simulink model "controllo_Completo_v14"  (R2025a)
settings: Solver=VariableStepAuto  StartTime=0.0  StopTime=Durata_Simulazione  MaxStep=Passo_integrazione_massimo  RelTol=1e-3
values from neighbouring files (symbols this model uses):
  C_bat_eq_rx = 1.0    (= 1)    [p_schema_completo_generale_v2.m]
  C_bat_eq_tx = 3.5    [p_schema_completo_generale_v2.m]
  C_bus_dc_dc = 1.5e-3    (= 0.0015)    [p_schema_completo_generale_v2.m]
  C_ris = 1/(w_dc_ac_nom^2*L_coil)    (= 6.49245057301e-08)    [p_schema_completo_generale_v2.m]
  dead_time_dc_dc = 0.3e-6    (= 3e-07)    [p_schema_completo_generale_v2.m]
  duty_A_0_tx = V_bat_0_tx/V_dc_0_tx    (= 0.472727272727)    [p_schema_completo_generale_v2.m]
  duty_B_0_tx = duty_A_0_tx    (= 0.472727272727)    [p_schema_completo_generale_v2.m]
  duty_leg_A_dc_dc_0_tx = V_bat_0_tx/V_dc_0_tx    (= 0.472727272727)    [p_schema_completo_generale_v2.m]
  duty_leg_B_dc_dc_0_tx = duty_leg_A_dc_dc_0_tx    (= 0.472727272727)    [p_schema_completo_generale_v2.m]
  Ibat_rif_max = 50    [p_schema_completo_generale_v2.m]
  Ibat_rif_min = -50    [p_schema_completo_generale_v2.m]
  Kp_P_tensione_batteria_rx = 1/modulo_catena_aperta_tensione_batteria_reg_P_rx    [p_schema_completo_generale_v2.m]
  Kp_P_tensione_batteria_tx = 1/modulo_catena_aperta_tensione_batteria_reg_P_tx    [p_schema_completo_generale_v2.m]
  L_coil = 54e-6    (= 5.4e-05)    [p_schema_completo_generale_v2.m]
  L_filtro_dc_dc = 65e-6    (= 6.5e-05)    [p_schema_completo_generale_v2.m]
  M_coil = k*sqrt(L_coil^2)    [p_schema_completo_generale_v2.m]
  Parametri_Controllori = [Parametri_Controllori     PI_corrente_trasm_tf_disc_den(2) PI_corrente_trasm_tf_disc_num(1) PI_corrente_trasm_tf_disc_num(2)]    [p_schema_completo_generale_v2.m]
  R_bat = 32e-3    (= 0.032)    [p_schema_completo_generale_v2.m]
  R_coil = w_dc_ac_nom*L_coil/Q_coil    (= 0.2883982056)    [p_schema_completo_generale_v2.m]
  R_coil_M = sqrt(w_dc_ac_nom^2)*M_coil/sqrt(Q_coil^2)    [p_schema_completo_generale_v2.m]
  R_Lfiltro_dc_dc = 6.5e-3    (= 0.0065)    [p_schema_completo_generale_v2.m]
  Req_Lfiltro_dc_dc = (R_Lfiltro_dc_dc+Rds_on_dc_dc)    (= 0.0075)    [p_schema_completo_generale_v2.m]
  Rshunt_coil = 1e5    (= 100000)    [p_schema_completo_generale_v2.m]
  Rshunt_Lfiltro = 1e6    (= 1000000)    [p_schema_completo_generale_v2.m]
  T_dc_ac = 1/freq_dc_ac    (= 1.17647058824e-05)    [p_schema_completo_generale_v2.m]
  T_dc_dc = 1/freq_dc_dc    (= 7.8431372549e-06)    [p_schema_completo_generale_v2.m]
  tau_filtro_anti_aliasing = R_filtro_anti_aliasing*C_filtro_anti_aliasing    (= 1.96e-06)    [p_schema_completo_generale_v2.m]
  tau_filtro_pb_coil = 1/(2*pi*f_filtro_pb_coil)    (= 3.18309886184e-05)    [p_schema_completo_generale_v2.m]
  tau_filtro_pb_corrente_bat = 1/(2*pi*f_filtro_pb_corrente_bat)    (= 2.49654812693e-05)    [p_schema_completo_generale_v2.m]
  Ts_BMS = 1e-3    (= 0.001)    [p_schema_completo_generale_v2.m]
  Ts_dc_ac = 4*T_dc_ac    (= 4.70588235294e-05)    [p_schema_completo_generale_v2.m]
  Ts_dc_dc = Ts_dc_ac    (= 4.70588235294e-05)    [p_schema_completo_generale_v2.m]
  Ts_trasmissione = 1e-3    (= 0.001)    [p_schema_completo_generale_v2.m]
  V_bat_0_rx = V_bat_nom    (= 96)    [p_schema_completo_generale_v2.m]
  V_bat_0_tx = V_bat_max-5    (= 104)    [p_schema_completo_generale_v2.m]
  V_bat_max = 109    [p_schema_completo_generale_v2.m]
  V_bat_max_alg = 218    [Controllo_tensione_bus_dc.m]    (also in Controllo_tensione_bus_dc_corrente_bobina.m; p_schema_completo_generale_v2.m)
  V_bat_min = 75    [p_schema_completo_generale_v2.m]
  V_bat_min_alg = 37.5    [Controllo_tensione_bus_dc.m]    (also in Controllo_tensione_bus_dc_corrente_bobina.m; p_schema_completo_generale_v2.m)
  V_dc_0_rx = 230    [p_schema_completo_generale_v2.m]
  V_dc_0_tx = 220    [p_schema_completo_generale_v2.m]
  Vbat_rif_max_tx = V_bat_max    (= 109)    [p_schema_completo_generale_v2.m]
  Vbat_rif_min_tx = V_bat_min    (= 75)    [p_schema_completo_generale_v2.m]
  Vdc_rif_max_tx = V_dc_nom+5    (= 255)    [p_schema_completo_generale_v2.m]
  Vdc_rif_min_tx = V_dc_nom-5    (= 245)    [p_schema_completo_generale_v2.m]
undefined symbols (not defined in the file or in its folder): Ceq_bat_tx, Cris_tx, Lfilt_dc_dc, Lfiltro_dc_dc_tx, R_bat_rx, R_bat_tx
libraries: simulink x44, spsSeriesRLCBranchLib x36, spsCurrentMeasurementLib x20, spsMosfetLib x16, spsVoltageMeasurementLib x12, simulink_extras x4, spsControlledCurrentSourceLib x4, spsControlledVoltageSourceLib x4, spsDCVoltageSourceLib x2, spsMutualInductanceLib x1, spsGroundLib x1, sps_lib x1
(part 2 of 7)

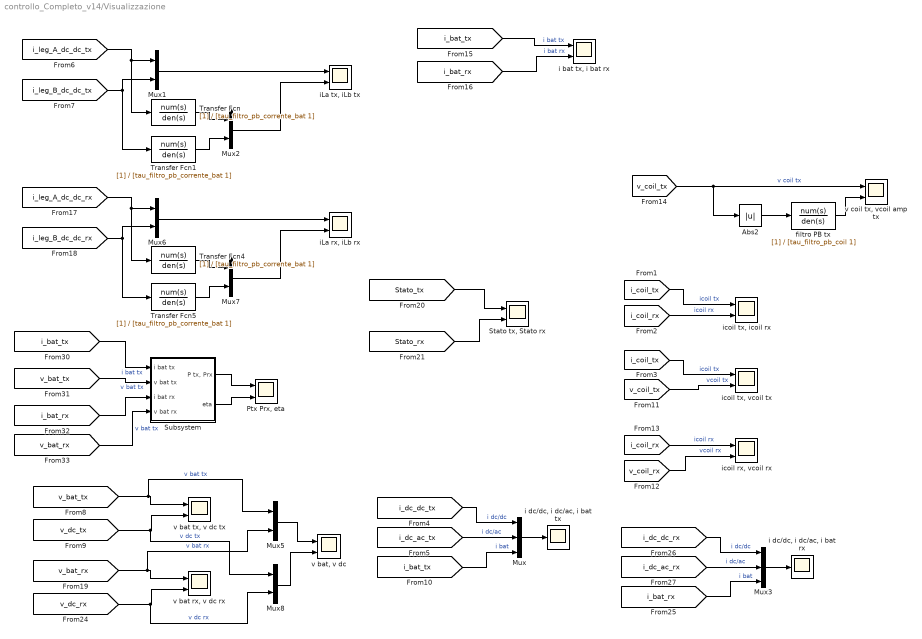
== system controllo_Completo_v14/Visualizzazione ==
  " Ptx Prx, eta" : Scope  NumInputPorts=2
      settings: ActiveDisplayYMinimum=-102.34489936147749  ActiveDisplayYMaximum=921.1040942532976  DataLoggingDecimation=10  DataLoggingVariableName=ScopeData20
  Abs2 : Abs  SaturateOnIntegerOverflow=off
  Mux : Mux  Inputs=3
  Mux{1..2,5..8} (6 alike) : Mux  Inputs=2
  Mux3 : Mux  Inputs=3
  "Stato tx, Stato rx" : Scope  NumInputPorts=2
      settings: ActiveDisplayYMinimum=0.28181818181818191  ActiveDisplayYMaximum=2.1909090909090909  DataLoggingDecimation=10  DataLoggingVariableName=ScopeData3
  Subsystem : Subsystem
  Transfer Fcn{,1,4..5} (4 alike) : TransferFcn  Denominator=[tau_filtro_pb_corrente_bat 1]
  filtro PB tx : TransferFcn  Denominator=[tau_filtro_pb_coil 1]
  "i bat tx, i bat rx" : Scope  NumInputPorts=2
      settings: ActiveDisplayYMinimum=-0.91269678315463987  ActiveDisplayYMaximum=8.2142710145221773  DataLoggingDecimation=10  DataLoggingVariableName=ScopeData31
  "i dc/dc, i dc/ac, i bat rx" : Scope
      settings: ActiveDisplayYMinimum=-50.858624395878969  ActiveDisplayYMaximum=5.6509582662087734  DataLoggingDecimation=10  DataLoggingVariableName=ScopeData41
  "i dc/dc, i dc/ac, i bat tx" : Scope
      settings: ActiveDisplayYMinimum=-4.661996714422445  ActiveDisplayYMaximum=41.953370131576783  DataLoggingDecimation=10
  "iLa rx, iLb rx" : Scope  NumInputPorts=2
      settings: ActiveDisplayYMinimum=-1.7782922823233973  ActiveDisplayYMaximum=0.19758803136926692  DataLoggingDecimation=10  DataLoggingVariableName=ScopeData34
  "iLa tx, iLb tx" : Scope  NumInputPorts=2
      settings: ActiveDisplayYMinimum=-0.98227394319739381  ActiveDisplayYMaximum=8.8404641169493079  DataLoggingDecimation=10
  "icoil rx, vcoil rx" : Scope  NumInputPorts=2
      settings: ActiveDisplayYMinimum=-2.9743876953698916  ActiveDisplayYMaximum=3.4975247511888838  DataLoggingDecimation=10  DataLoggingVariableName=ScopeData33
  "icoil tx, icoil rx" : Scope  NumInputPorts=2
      settings: ActiveDisplayYMinimum=-59.257229970690162  ActiveDisplayYMaximum=60.524143535599663  DataLoggingDecimation=10  DataLoggingVariableName=ScopeData30
  "icoil tx, vcoil tx" : Scope  NumInputPorts=2
      settings: ActiveDisplayYMinimum=-54.3619489771676  ActiveDisplayYMaximum=54.345891292400964  DataLoggingDecimation=10  DataLoggingVariableName=ScopeData32
  "v bat rx, v dc rx" : Scope  NumInputPorts=2
      settings: ActiveDisplayYMinimum=85.572933342877334  ActiveDisplayYMaximum=97.158562961902518  DataLoggingDecimation=10  DataLoggingVariableName=ScopeData36
  "v bat tx, v dc tx" : Scope  NumInputPorts=2
      settings: ActiveDisplayYMinimum=226.74014486787908  ActiveDisplayYMaximum=259.31993544703744  DataLoggingDecimation=10  DataLoggingVariableName=ScopeData2
  "v bat, v dc" : Scope  NumInputPorts=2
      settings: ActiveDisplayYMinimum=94.999999999276838  ActiveDisplayYMaximum=105.00000000647344  DataLoggingDecimation=10  DataLoggingVariableName=ScopeData10
  "v coil tx, vcoil amp tx" : Scope  NumInputPorts=2
      settings: ActiveDisplayYMinimum=-320.06773075412292  ActiveDisplayYMaximum=320.06780035221288  DataLoggingDecimation=10  DataLoggingVariableName=ScopeData23
  wires:
  [Stato_rx] -> "Stato tx, Stato rx"/2
  [Stato_tx] -> "Stato tx, Stato rx"/1
  Subsystem/2(eta) -> " Ptx Prx, eta"/2
  Subsystem/1("P tx, Prx") -> " Ptx Prx, eta"/1
  [v_bat_rx] -> Subsystem/4(v bat rx)  "v bat tx"
  [i_bat_rx] -> Subsystem/3(i bat rx)
  [v_bat_tx] -> Subsystem/2(v bat tx)  "v bat tx"
  [i_bat_tx] -> Subsystem/1(i bat tx)  "i bat tx"
  Mux5/1 -> "v bat, v dc"/1
  Mux8/1 -> "v bat, v dc"/2
  Mux3/1 -> "i dc/dc, i dc/ac, i bat rx"/1
  [i_bat_rx] -> Mux3/3  "i bat"
  [i_dc_dc_rx] -> Mux3/1  "i dc/dc"
  [i_dc_ac_rx] -> Mux3/2  "i dc/ac"
  [v_dc_rx] -> "v bat rx, v dc rx"/2, Mux8/2  "v dc rx"
  [v_bat_rx] -> "v bat rx, v dc rx"/1, Mux5/2  "v bat rx"
  [i_bat_rx] -> "i bat tx, i bat rx"/2  "i bat rx"
  [i_bat_tx] -> "i bat tx, i bat rx"/1  "i bat tx"
  Transfer Fcn4/1 -> Mux7/1
  [i_leg_B_dc_dc_rx] -> Mux6/2, Transfer Fcn5/1
  Mux6/1 -> "iLa rx, iLb rx"/1
  [i_leg_A_dc_dc_rx] -> Transfer Fcn4/1, Mux6/1
  Transfer Fcn5/1 -> Mux7/2
  Mux7/1 -> "iLa rx, iLb rx"/2
  Abs2/1 -> filtro PB tx/1
  [v_coil_tx] -> "v coil tx, vcoil amp tx"/1, Abs2/1  "v coil tx"
  filtro PB tx/1 -> "v coil tx, vcoil amp tx"/2
  [i_coil_rx] -> "icoil rx, vcoil rx"/1  "icoil rx"
  [v_coil_rx] -> "icoil rx, vcoil rx"/2  "vcoil rx"
  [i_coil_tx] -> "icoil tx, vcoil tx"/1  "icoil tx"
  [v_coil_tx] -> "icoil tx, vcoil tx"/2  "vcoil tx"
  [i_coil_rx] -> "icoil tx, icoil rx"/2  "icoil rx"
  [i_coil_tx] -> "icoil tx, icoil rx"/1  "icoil tx"
  Mux2/1 -> "iLa tx, iLb tx"/2
  [i_dc_ac_tx] -> Mux/2  "i dc/ac"
  Mux1/1 -> "iLa tx, iLb tx"/1
  [i_dc_dc_tx] -> Mux/1  "i dc/dc"
  Transfer Fcn/1 -> Mux2/1
  Transfer Fcn1/1 -> Mux2/2
  Mux/1 -> "i dc/dc, i dc/ac, i bat tx"/1
  [v_bat_tx] -> "v bat tx, v dc tx"/1, Mux5/1  "v bat tx"
  [i_leg_A_dc_dc_tx] -> Transfer Fcn/1, Mux1/1
  [i_leg_B_dc_dc_tx] -> Mux1/2, Transfer Fcn1/1
  [i_bat_tx] -> Mux/3  "i bat"
  [v_dc_tx] -> "v bat tx, v dc tx"/2, Mux8/1  "v dc tx"

== system controllo_Completo_v14/Batteria/Batteria ==
  DC Voltage Source : spsDCVoltageSourceLib/DC Voltage Source  Amplitude=V_bat_0_tx  Measurements=None
  Series RLC Branch1 : spsSeriesRLCBranchLib/Series RLC Branch  LConnTagsString=__new0  RConnTagsString=__new0  BranchType=R  Resistance=R_bat_tx  Inductance=1e-3  SetiL0=off  InitialCurrent=0  Capacitance=1e-6  Setx0=off  InitialVoltage=0  Measurements=None
  Vbat tx : PMIOPort  Side=Right
  Vgnd tx : PMIOPort  Port=2  Side=Right
  connections:
  Vgnd tx/RConn1 -- DC Voltage Source/LConn1
  DC Voltage Source/RConn1 -- Series RLC Branch1/RConn1
  Vbat tx/RConn1 -- Series RLC Branch1/LConn1

== system controllo_Completo_v14/Batteria/Condensatore ==
  Series RLC Branch : spsSeriesRLCBranchLib/Series RLC Branch  LConnTagsString=__new0  RConnTagsString=__new0  BranchType=C  Resistance=1  Inductance=Ceq_bat_tx  SetiL0=off  InitialCurrent=0  Capacitance=C_bat_eq_tx  Setx0=on  InitialVoltage=V_bat_0_tx  Measurements=None
  Series RLC Branch1 : spsSeriesRLCBranchLib/Series RLC Branch  LConnTagsString=__new0  RConnTagsString=__new0  BranchType=R  Resistance=R_bat  Inductance=1e-3  SetiL0=off  InitialCurrent=0  Capacitance=1e-6  Setx0=off  InitialVoltage=0  Measurements=None
  Vbat tx : PMIOPort  Side=Right
  Vgnd tx : PMIOPort  Port=2  Side=Right
  connections:
  Series RLC Branch/LConn1 -- Series RLC Branch1/RConn1
  Vbat tx/RConn1 -- Series RLC Branch1/LConn1
  Vgnd tx/RConn1 -- Series RLC Branch/RConn1

== system controllo_Completo_v14/Batteria /Batteria ==
  DC Voltage Source : spsDCVoltageSourceLib/DC Voltage Source  Amplitude=V_bat_0_rx  Measurements=None
  Series RLC Branch1 : spsSeriesRLCBranchLib/Series RLC Branch  LConnTagsString=__new0  RConnTagsString=__new0  BranchType=R  Resistance=R_bat_rx  Inductance=1e-3  SetiL0=off  InitialCurrent=0  Capacitance=1e-6  Setx0=off  InitialVoltage=0  Measurements=None
  Vbat rx : PMIOPort  Side=Right
  Vgnd rx : PMIOPort  Port=2  Side=Right
  connections:
  Vgnd rx/RConn1 -- DC Voltage Source/LConn1
  DC Voltage Source/RConn1 -- Series RLC Branch1/RConn1
  Vbat rx/RConn1 -- Series RLC Branch1/LConn1

== system controllo_Completo_v14/Batteria /Condensatore ==
  Series RLC Branch : spsSeriesRLCBranchLib/Series RLC Branch  LConnTagsString=__new0  RConnTagsString=__new0  BranchType=C  Resistance=1  Inductance=Ceq_bat_tx  SetiL0=off  InitialCurrent=0  Capacitance=C_bat_eq_rx  Setx0=on  InitialVoltage=V_bat_0_rx  Measurements=None
  Series RLC Branch1 : spsSeriesRLCBranchLib/Series RLC Branch  LConnTagsString=__new0  RConnTagsString=__new0  BranchType=R  Resistance=R_bat  Inductance=1e-3  SetiL0=off  InitialCurrent=0  Capacitance=1e-6  Setx0=off  InitialVoltage=0  Measurements=None
  Vbat rx : PMIOPort  Side=Right
  Vgnd rx : PMIOPort  Port=2  Side=Right
  connections:
  Series RLC Branch/LConn1 -- Series RLC Branch1/RConn1
  Vbat rx/RConn1 -- Series RLC Branch1/LConn1
  Vgnd rx/RConn1 -- Series RLC Branch/RConn1

== system controllo_Completo_v14/Controllo  rx/Modulazione PS ==
  duty A : Inport
  duty B : Inport  Port=2
  abilita PWM : Inport  Port=3
  Dead time : Subsystem  Variant=on
  Phase shift : Subsystem
  high A DT : Outport
  low A DT : Outport  Port=2
  high B DT : Outport  Port=3
  low B DT : Outport  Port=4
  wires:
  Phase shift/1(high A) -> Dead time/1(high A)
  Dead time/4(low B DT) -> low B DT/1
  Dead time/2(low A DT) -> low A DT/1
  Phase shift/3(high B) -> Dead time/3(high B)
  duty A/1 -> Phase shift/1(duty A)
  Phase shift/4(low B) -> Dead time/4(low B)
  Phase shift/2(low A) -> Dead time/2(low A)
  Dead time/3(high B DT) -> high B DT/1
  duty B/1 -> Phase shift/2(duty B)
  Dead time/1(high A DT) -> high A DT/1
  abilita PWM/1 -> Phase shift/3(abilita PWM)

== system controllo_Completo_v14/Controllo  rx/Modulazione PWM ==
  duty A : Inport
  duty B : Inport  Port=2
  abilita PWM : Inport  Port=3
  Variant Subsystem : Subsystem  Variant=on
  Variant Subsystem1 : Subsystem  Variant=on
  high A dead time / duty A : Outport
  low A dead time : Outport  Port=2
  high B dead time / duty B : Outport  Port=3
  low B dead time : Outport  Port=4
  wires:
  abilita PWM/1 -> Variant Subsystem1/3(abilita PWM)
  Variant Subsystem/4(low B DT) -> low B dead time/1
  Variant Subsystem/3(high B DT) -> high B dead time / duty B/1
  Variant Subsystem/2(low A DT) -> low A dead time/1
  Variant Subsystem/1(high A DT) -> high A dead time / duty A/1
  duty A/1 -> Variant Subsystem1/1(duty A)
  Variant Subsystem1/3(high B) -> Variant Subsystem/3(high B)
  Variant Subsystem1/2(low A) -> Variant Subsystem/2(low A)
  duty B/1 -> Variant Subsystem1/2(duty B)
  Variant Subsystem1/1(high A) -> Variant Subsystem/1(high A)
  Variant Subsystem1/4(low B) -> Variant Subsystem/4(low B)

== system controllo_Completo_v14/Controllo tx/Modulazione PS ==
  duty A : Inport
  duty B : Inport  Port=2
  abilita PWM : Inport  Port=3
  Dead time : Subsystem  Variant=on
  Phase shift : Subsystem
  high A DT : Outport
  low A DT : Outport  Port=2
  high B DT : Outport  Port=3
  low B DT : Outport  Port=4
  wires:
  Phase shift/1(high A) -> Dead time/1(high A)
  Dead time/4(low B DT) -> low B DT/1
  Dead time/2(low A DT) -> low A DT/1
  Phase shift/3(high B) -> Dead time/3(high B)
  duty A/1 -> Phase shift/1(duty A)
  Phase shift/4(low B) -> Dead time/4(low B)
  Phase shift/2(low A) -> Dead time/2(low A)
  Dead time/3(high B DT) -> high B DT/1
  duty B/1 -> Phase shift/2(duty B)
  Dead time/1(high A DT) -> high A DT/1
  abilita PWM/1 -> Phase shift/3(abilita PWM)

== system controllo_Completo_v14/Controllo tx/Modulazione PWM ==
  duty A : Inport
  duty B : Inport  Port=2
  abilita PWM : Inport  Port=3
  Variant Subsystem : Subsystem  Variant=on
  Variant Subsystem1 : Subsystem  Variant=on
  high A dead time / duty A : Outport
  low A dead time : Outport  Port=2
  high B dead time / duty B : Outport  Port=3
  low B dead time : Outport  Port=4
  wires:
  Variant Subsystem1/4(low B) -> Variant Subsystem/4(low B)
  Variant Subsystem1/1(high A) -> Variant Subsystem/1(high A)
  duty B/1 -> Variant Subsystem1/2(duty B)
  Variant Subsystem1/2(low A) -> Variant Subsystem/2(low A)
  Variant Subsystem1/3(high B) -> Variant Subsystem/3(high B)
  duty A/1 -> Variant Subsystem1/1(duty A)
  Variant Subsystem/1(high A DT) -> high A dead time / duty A/1
  Variant Subsystem/2(low A DT) -> low A dead time/1
  Variant Subsystem/3(high B DT) -> high B dead time / duty B/1
  Variant Subsystem/4(low B DT) -> low B dead time/1
  abilita PWM/1 -> Variant Subsystem1/3(abilita PWM)

== system controllo_Completo_v14/Convertitore dc-dc/Convertitore dc-dc switching ==
  note: Tx
  Current Measurement{,1..2,4} (4 alike) : spsCurrentMeasurementLib/Current Measurement  PhasorSimulation=off  OutputType=Complex  PSBequivalent=0
  Goto4 : Goto  Commented=on  GotoTag=v_dc_tx  TagVisibility=global
  Mosfet{,1..3} (4 alike) : spsMosfetLib/Mosfet  Ron=Rds_on_dc_dc  Lon=0  Rd=Ron_diodo_dc_dc  Vfd=Vf_diodo_dc_dc  IC=0  Rs=Rsnubber_dc_dc  Cs=Csnubber_dc_dc  Measurements=off
  Series RLC Branch1 : spsSeriesRLCBranchLib/Series RLC Branch  LConnTagsString=__new0  RConnTagsString=__new0  BranchType=R  Resistance=Rshunt_Lfiltro  Inductance=Lfiltro_dc_dc_tx  SetiL0=on  InitialCurrent=Imedia_bat_B_tx  Capacitance=1e-6  Setx0=off  InitialVoltage=0  Measurements=None
  Series RLC Branch2 : spsSeriesRLCBranchLib/Series RLC Branch  LConnTagsString=__new0  RConnTagsString=__new0  BranchType=R  Resistance=Rshunt_Lfiltro  Inductance=Lfiltro_dc_dc_tx  SetiL0=on  InitialCurrent=Imedia_bat_B_tx  Capacitance=1e-6  Setx0=off  InitialVoltage=0  Measurements=None
  Series RLC Branch3 : spsSeriesRLCBranchLib/Series RLC Branch  LConnTagsString=__new0  RConnTagsString=__new0  BranchType=R  Resistance=R_Lfiltro_dc_dc  Inductance=Lfiltro_dc_dc_tx  SetiL0=on  InitialCurrent=Imedia_bat_B_tx  Capacitance=1e-6  Setx0=off  InitialVoltage=0  Measurements=None
  Series RLC Branch4 : spsSeriesRLCBranchLib/Series RLC Branch  LConnTagsString=__new0  RConnTagsString=__new0  BranchType=R  Resistance=R_Lfiltro_dc_dc  Inductance=Lfiltro_dc_dc_tx  SetiL0=on  InitialCurrent=Imedia_bat_B_tx  Capacitance=1e-6  Setx0=off  InitialVoltage=0  Measurements=None
  Series RLC Branch5 : spsSeriesRLCBranchLib/Series RLC Branch  LConnTagsString=__new0  RConnTagsString=__new0  BranchType=L  Resistance=1  Inductance=L_filtro_dc_dc  SetiL0=on  InitialCurrent=I_Lfiltro_B_0_tx  Capacitance=1e-6  Setx0=off  InitialVoltage=0  Measurements=None
  Series RLC Branch6 : spsSeriesRLCBranchLib/Series RLC Branch  LConnTagsString=__new0  RConnTagsString=__new0  BranchType=L  Resistance=1  Inductance=L_filtro_dc_dc  SetiL0=on  InitialCurrent=I_Lfiltro_A_0_tx  Capacitance=1e-6  Setx0=off  InitialVoltage=0  Measurements=None
  Voltage Measurement : spsVoltageMeasurementLib/Voltage Measurement  Commented=on  PhasorSimulation=off  OutputType=Complex  PSBequivalent=0
  Voltage Measurement1 : spsVoltageMeasurementLib/Voltage Measurement  PhasorSimulation=off  OutputType=Complex  PSBequivalent=0
  Vdc tx : PMIOPort  Side=Right
  Vgnd tx : PMIOPort  Port=2  Side=Right
  Vbat + tx : PMIOPort  Port=3  Side=Left
  Vbat - tx : PMIOPort  Port=4  Side=Left
  tag scope: i_bat_tx=global, i_dc_dc_tx=global, i_leg_A_dc_dc_tx=global, i_leg_B_dc_dc_tx=global, v_bat_tx=global
  wires:
  Current Measurement/1 -> [i_leg_B_dc_dc_tx]
  [dc_dc_leg_B_low_tx] -> Mosfet3/1
  [dc_dc_leg_A_low_tx] -> Mosfet1/1
  [dc_dc_leg_A_high_tx] -> Mosfet/1
  [dc_dc_leg_B_high_tx] -> Mosfet2/1
  Current Measurement1/1 -> [i_leg_A_dc_dc_tx]
  Current Measurement2/1 -> [i_dc_dc_tx]
  Voltage Measurement1/1 -> [v_bat_tx]
  Voltage Measurement/1 -> Goto4/1
  Current Measurement4/1 -> [i_bat_tx]
  connections:
  Current Measurement2/LConn1 -- Mosfet2/LConn1 -- Mosfet/LConn1
  Mosfet3/RConn1 -- Vgnd tx/RConn1 -- Voltage Measurement/LConn2 -- Mosfet1/RConn1 -- Vbat - tx/RConn1 -- Voltage Measurement1/LConn2
  Voltage Measurement1/LConn1 -- Vbat + tx/RConn1 -- Current Measurement4/LConn1
  Series RLC Branch3/RConn1 -- Mosfet1/LConn1 -- Mosfet/RConn1
  Series RLC Branch2/LConn1 -- Series RLC Branch6/LConn1 -- Current Measurement1/RConn1
  Series RLC Branch1/LConn1 -- Series RLC Branch5/LConn1 -- Current Measurement/RConn1
  Series RLC Branch2/RConn1 -- Series RLC Branch3/LConn1 -- Series RLC Branch6/RConn1
  Series RLC Branch5/RConn1 -- Series RLC Branch4/LConn1 -- Series RLC Branch1/RConn1
  Series RLC Branch4/RConn1 -- Mosfet2/RConn1 -- Mosfet3/LConn1
  Current Measurement/LConn1 -- Current Measurement1/LConn1 -- Current Measurement4/RConn1
  Voltage Measurement/LConn1 -- Current Measurement2/RConn1 -- Vdc tx/RConn1

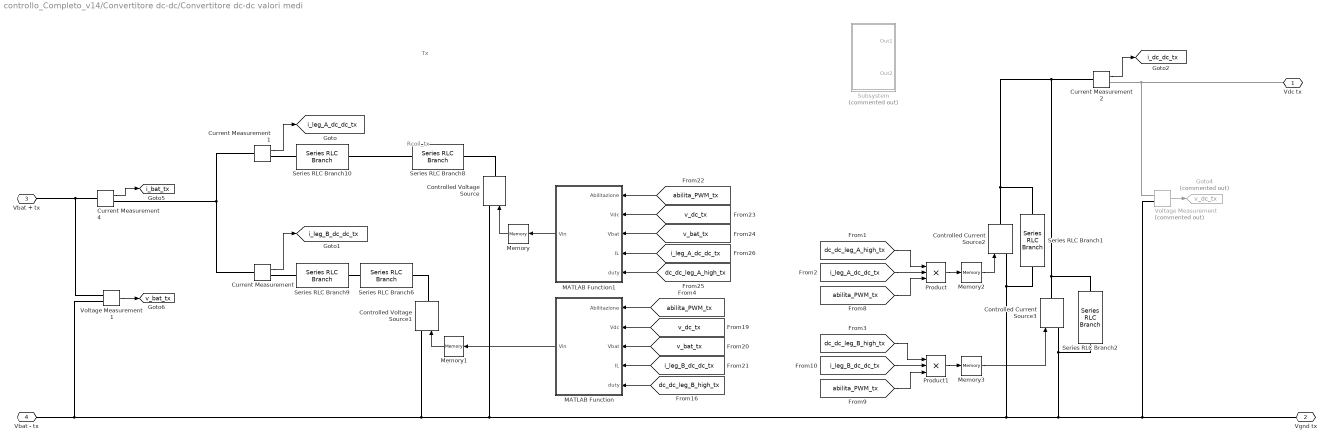
== system controllo_Completo_v14/Convertitore dc-dc/Convertitore dc-dc valori medi ==
  note: Rcoil_tx
  note: Tx
  Controlled Current Source2 : spsControlledCurrentSourceLib/Controlled Current Source  Initialize=on  Source_Type=AC  Amplitude=0  Phase=0  Frequency=0  Measurements=None
  Controlled Current Source3 : spsControlledCurrentSourceLib/Controlled Current Source  Initialize=on  Source_Type=AC  Amplitude=0  Phase=0  Frequency=0  Measurements=None
  Controlled Voltage Source : spsControlledVoltageSourceLib/Controlled Voltage Source  Initialize=on  Source_Type=DC  Amplitude=duty_leg_A_dc_dc_0_tx*V_dc_0_tx  Phase=0  Frequency=0  Measurements=None
  Controlled Voltage Source1 : spsControlledVoltageSourceLib/Controlled Voltage Source  Initialize=on  Source_Type=DC  Amplitude=duty_leg_B_dc_dc_0_tx*V_dc_0_tx  Phase=0  Frequency=0  Measurements=None
  Current Measurement{,1..2,4} (4 alike) : spsCurrentMeasurementLib/Current Measurement  PhasorSimulation=off  OutputType=Complex  PSBequivalent=0
  Goto4 : Goto  Commented=on  GotoTag=v_dc_tx  TagVisibility=global
  MATLAB Function : MATLAB Function  TreatAsAtomicUnit=on
  MATLAB Function1 : MATLAB Function  TreatAsAtomicUnit=on
  Memory{,1..3} (4 alike) : Memory
  Product : Product  Inputs=3
  Product1 : Product  Inputs=3
  Series RLC Branch1 : spsSeriesRLCBranchLib/Series RLC Branch  LConnTagsString=__new0  RConnTagsString=__new0  BranchType=R  Resistance=Rshunt_Lfiltro  Inductance=Lfiltro_dc_dc_tx  SetiL0=on  InitialCurrent=Imedia_bat_B_tx  Capacitance=1e-6  Setx0=off  InitialVoltage=0  Measurements=None
  Series RLC Branch10 : spsSeriesRLCBranchLib/Series RLC Branch  LConnTagsString=__new0  RConnTagsString=__new0  BranchType=L  Resistance=1  Inductance=L_filtro_dc_dc  SetiL0=off  InitialCurrent=I_Lfiltro_A_0_tx  Capacitance=1e-6  Setx0=off  InitialVoltage=0  Measurements=None
  Series RLC Branch2 : spsSeriesRLCBranchLib/Series RLC Branch  LConnTagsString=__new0  RConnTagsString=__new0  BranchType=R  Resistance=Rshunt_Lfiltro  Inductance=Lfiltro_dc_dc_tx  SetiL0=on  InitialCurrent=Imedia_bat_B_tx  Capacitance=1e-6  Setx0=off  InitialVoltage=0  Measurements=None
  Series RLC Branch6 : spsSeriesRLCBranchLib/Series RLC Branch  LConnTagsString=__new0  RConnTagsString=__new0  BranchType=R  Resistance=Req_Lfiltro_dc_dc  Inductance=Lfiltro_dc_dc_tx  SetiL0=on  InitialCurrent=Imedia_bat_B_tx  Capacitance=1e-6  Setx0=off  InitialVoltage=0  Measurements=None
  Series RLC Branch8 : spsSeriesRLCBranchLib/Series RLC Branch  LConnTagsString=__new0  RConnTagsString=__new0  BranchType=R  Resistance=Req_Lfiltro_dc_dc  Inductance=Lfiltro_dc_dc_tx  SetiL0=on  InitialCurrent=Imedia_bat_B_tx  Capacitance=1e-6  Setx0=off  InitialVoltage=0  Measurements=None
  Series RLC Branch9 : spsSeriesRLCBranchLib/Series RLC Branch  LConnTagsString=__new0  RConnTagsString=__new0  BranchType=L  Resistance=1  Inductance=L_filtro_dc_dc  SetiL0=off  InitialCurrent=I_Lfiltro_B_0_tx  Capacitance=1e-6  Setx0=off  InitialVoltage=0  Measurements=None
  Subsystem : Subsystem  Commented=on
  Voltage Measurement : spsVoltageMeasurementLib/Voltage Measurement  Commented=on  PhasorSimulation=off  OutputType=Complex  PSBequivalent=0
  Voltage Measurement1 : spsVoltageMeasurementLib/Voltage Measurement  PhasorSimulation=off  OutputType=Complex  PSBequivalent=0
  Vdc tx : PMIOPort  Side=Right
  Vgnd tx : PMIOPort  Port=2  Side=Right
  Vbat + tx : PMIOPort  Port=3  Side=Left
  Vbat - tx : PMIOPort  Port=4  Side=Left
  tag scope: i_bat_tx=global, i_dc_dc_tx=global, i_leg_A_dc_dc_tx=global, i_leg_B_dc_dc_tx=global, v_bat_tx=global
  wires:
  Current Measurement1/1 -> [i_leg_A_dc_dc_tx]
  Current Measurement2/1 -> [i_dc_dc_tx]
  Memory3/1 -> Controlled Current Source3/1
  Memory/1 -> Controlled Voltage Source/1
  Voltage Measurement/1 -> Goto4/1
  [dc_dc_leg_A_high_tx] -> Product/1
  Product1/1 -> Memory3/1
  [i_leg_A_dc_dc_tx] -> Product/2
  Memory2/1 -> Controlled Current Source2/1
  Current Measurement/1 -> [i_leg_B_dc_dc_tx]
  [dc_dc_leg_B_high_tx] -> Product1/1
  Current Measurement4/1 -> [i_bat_tx]
  Product/1 -> Memory2/1
  [i_leg_B_dc_dc_tx] -> Product1/2
  Memory1/1 -> Controlled Voltage Source1/1
  Voltage Measurement1/1 -> [v_bat_tx]
  [abilita_PWM_tx] -> Product/3
  [abilita_PWM_tx] -> Product1/3
  [abilita_PWM_tx] -> MATLAB Function/1(Abilitazione)
  [dc_dc_leg_B_high_tx] -> MATLAB Function/5(duty)
  [v_dc_tx] -> MATLAB Function/2(Vdc)
  [v_bat_tx] -> MATLAB Function/3(Vbat)
  [i_leg_B_dc_dc_tx] -> MATLAB Function/4(IL)
  MATLAB Function/1(Vin) -> Memory1/1
  [abilita_PWM_tx] -> MATLAB Function1/1(Abilitazione)
  [v_dc_tx] -> MATLAB Function1/2(Vdc)
  [v_bat_tx] -> MATLAB Function1/3(Vbat)
  [dc_dc_leg_A_high_tx] -> MATLAB Function1/5(duty)
  [i_leg_A_dc_dc_tx] -> MATLAB Function1/4(IL)
  MATLAB Function1/1(Vin) -> Memory/1
  connections:
  Voltage Measurement/LConn1 -- Current Measurement2/RConn1 -- Vdc tx/RConn1
  Controlled Voltage Source/LConn1 -- Series RLC Branch2/RConn1 -- Controlled Current Source3/LConn1 -- Vgnd tx/RConn1 -- Voltage Measurement/LConn2 -- Series RLC Branch1/RConn1 -- Controlled Current Source2/LConn1 -- Controlled Voltage Source1/LConn1 -- Vbat - tx/RConn1 -- Voltage Measurement1/LConn2
  Current Measurement4/RConn1 -- Current Measurement/LConn1 -- Current Measurement1/LConn1
  Current Measurement4/LConn1 -- Vbat + tx/RConn1 -- Voltage Measurement1/LConn1
  Controlled Current Source3/RConn1 -- Series RLC Branch1/LConn1 -- Controlled Current Source2/RConn1 -- Current Measurement2/LConn1 -- Series RLC Branch2/LConn1
  Controlled Voltage Source/RConn1 -- Series RLC Branch8/RConn1
  Series RLC Branch6/RConn1 -- Controlled Voltage Source1/RConn1
  Current Measurement/RConn1 -- Series RLC Branch9/LConn1
  Series RLC Branch6/LConn1 -- Series RLC Branch9/RConn1
  Series RLC Branch10/RConn1 -- Series RLC Branch8/LConn1
  Current Measurement1/RConn1 -- Series RLC Branch10/LConn1

== system controllo_Completo_v14/Convertitore dc-dc /Convertitore dc-dc Switching  ==
  note: Rx
  Current Measurement{,1..2,4} (4 alike) : spsCurrentMeasurementLib/Current Measurement  PhasorSimulation=off  OutputType=Complex  PSBequivalent=0
  Goto4 : Goto  Commented=on  GotoTag=v_dc_rx  TagVisibility=global
  Mosfet{1..4} (4 alike) : spsMosfetLib/Mosfet  Ron=Rds_on_dc_dc  Lon=0  Rd=Ron_diodo_dc_dc  Vfd=Vf_diodo_dc_dc  IC=0  Rs=Rsnubber_dc_dc  Cs=Csnubber_dc_dc  Measurements=on
  Series RLC Branch1 : spsSeriesRLCBranchLib/Series RLC Branch  LConnTagsString=__new0  RConnTagsString=__new0  BranchType=R  Resistance=Rshunt_Lfiltro  Inductance=Lfiltro_dc_dc_tx  SetiL0=on  InitialCurrent=Imedia_bat_B_tx  Capacitance=1e-6  Setx0=off  InitialVoltage=0  Measurements=None
  Series RLC Branch2 : spsSeriesRLCBranchLib/Series RLC Branch  Commented=on  LConnTagsString=__new0  RConnTagsString=__new0  BranchType=R  Resistance=Rshunt_Lfiltro  Inductance=Lfiltro_dc_dc_tx  SetiL0=on  InitialCurrent=Imedia_bat_B_tx  Capacitance=1e-6  Setx0=off  InitialVoltage=0  Measurements=None
  Series RLC Branch3 : spsSeriesRLCBranchLib/Series RLC Branch  LConnTagsString=__new0  RConnTagsString=__new0  BranchType=R  Resistance=R_Lfiltro_dc_dc  Inductance=Lfiltro_dc_dc_tx  SetiL0=on  InitialCurrent=Imedia_bat_B_tx  Capacitance=1e-6  Setx0=off  InitialVoltage=0  Measurements=None
  Series RLC Branch4 : spsSeriesRLCBranchLib/Series RLC Branch  LConnTagsString=__new0  RConnTagsString=__new0  BranchType=R  Resistance=R_Lfiltro_dc_dc  Inductance=Lfiltro_dc_dc_tx  SetiL0=on  InitialCurrent=Imedia_bat_B_tx  Capacitance=1e-6  Setx0=off  InitialVoltage=0  Measurements=None
  Series RLC Branch5 : spsSeriesRLCBranchLib/Series RLC Branch  LConnTagsString=__new0  RConnTagsString=__new0  BranchType=L  Resistance=1  Inductance=L_filtro_dc_dc  SetiL0=off  InitialCurrent=I_Lfiltro_B_0_rx  Capacitance=1e-6  Setx0=off  InitialVoltage=0  Measurements=None
  Series RLC Branch6 : spsSeriesRLCBranchLib/Series RLC Branch  LConnTagsString=__new0  RConnTagsString=__new0  BranchType=L  Resistance=1  Inductance=L_filtro_dc_dc  SetiL0=off  InitialCurrent=I_Lfiltro_A_0_rx  Capacitance=1e-6  Setx0=off  InitialVoltage=0  Measurements=None
  Voltage Measurement : spsVoltageMeasurementLib/Voltage Measurement  Commented=on  PhasorSimulation=off  OutputType=Complex  PSBequivalent=0
  Voltage Measurement1 : spsVoltageMeasurementLib/Voltage Measurement  PhasorSimulation=off  OutputType=Complex  PSBequivalent=0
  Vdc rx : PMIOPort  Side=Left
  "Vgnd rx " : PMIOPort  Port=2  Side=Left
  Vbat + rx : PMIOPort  Port=3  Side=Right
  Vbat - rx : PMIOPort  Port=4  Side=Right
  tag scope: i_bat_rx=global, i_dc_dc_rx=global, i_leg_A_dc_dc_rx=global, i_leg_B_dc_dc_rx=global, v_bat_rx=global
  wires:
  Current Measurement1/1 -> [i_leg_A_dc_dc_rx]
  Voltage Measurement1/1 -> [v_bat_rx]
  [dc_dc_leg_B_low_rx] -> Mosfet3/1
  [dc_dc_leg_A_low_rx] -> Mosfet1/1
  [dc_dc_leg_A_high_rx] -> Mosfet4/1
  Current Measurement4/1 -> [i_bat_rx]
  [dc_dc_leg_B_high_rx] -> Mosfet2/1
  Current Measurement/1 -> [i_leg_B_dc_dc_rx]
  Current Measurement2/1 -> [i_dc_dc_rx]
  Voltage Measurement/1 -> Goto4/1
  connections:
  Series RLC Branch4/RConn1 -- Mosfet2/RConn1 -- Mosfet3/LConn1
  Series RLC Branch1/LConn1 -- Current Measurement/RConn1 -- Series RLC Branch5/LConn1
  Voltage Measurement/LConn2 -- Mosfet1/RConn1 -- Vbat - rx/RConn1 -- Voltage Measurement1/LConn2 -- Mosfet3/RConn1 -- "Vgnd rx "/RConn1
  Series RLC Branch2/RConn1 -- Series RLC Branch6/RConn1 -- Series RLC Branch3/LConn1
  Voltage Measurement1/LConn1 -- Vbat + rx/RConn1 -- Current Measurement4/LConn1
  Current Measurement/LConn1 -- Current Measurement1/LConn1 -- Current Measurement4/RConn1
  Current Measurement2/RConn1 -- Voltage Measurement/LConn1 -- Vdc rx/RConn1
  Mosfet4/LConn1 -- Current Measurement2/LConn1 -- Mosfet2/LConn1
  Mosfet4/RConn1 -- Mosfet1/LConn1 -- Series RLC Branch3/RConn1
  Series RLC Branch5/RConn1 -- Series RLC Branch1/RConn1 -- Series RLC Branch4/LConn1
  Series RLC Branch2/LConn1 -- Current Measurement1/RConn1 -- Series RLC Branch6/LConn1

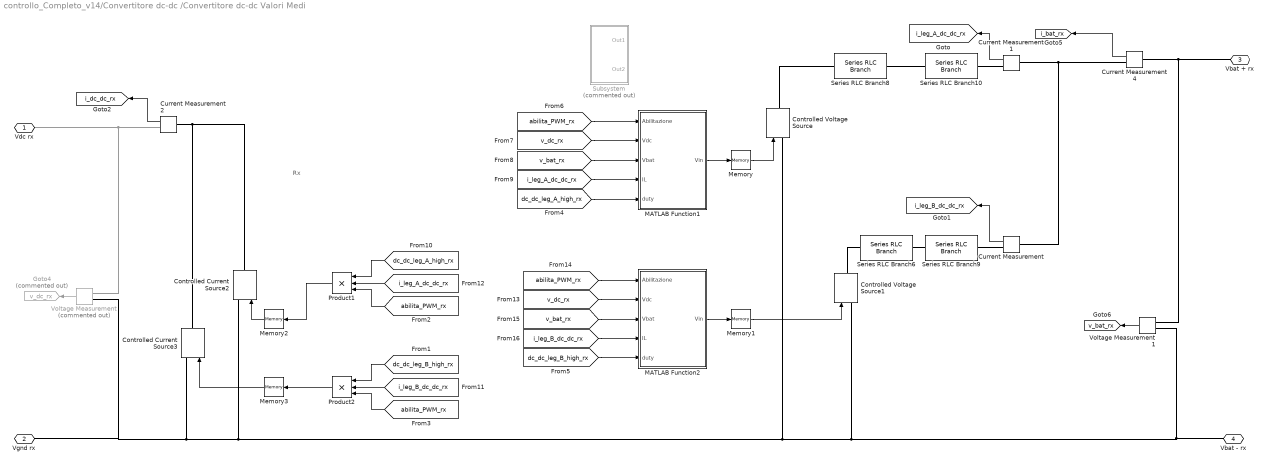
== system controllo_Completo_v14/Convertitore dc-dc /Convertitore dc-dc Valori Medi  ==
  note: Rx
  Controlled Current Source2 : spsControlledCurrentSourceLib/Controlled Current Source  Initialize=on  Source_Type=AC  Amplitude=0  Phase=0  Frequency=0  Measurements=None
  Controlled Current Source3 : spsControlledCurrentSourceLib/Controlled Current Source  Initialize=on  Source_Type=AC  Amplitude=0  Phase=0  Frequency=0  Measurements=None
  Controlled Voltage Source : spsControlledVoltageSourceLib/Controlled Voltage Source  Initialize=on  Source_Type=DC  Amplitude=duty_leg_A_dc_dc_0_tx*V_dc_0_rx  Phase=0  Frequency=0  Measurements=None
  Controlled Voltage Source1 : spsControlledVoltageSourceLib/Controlled Voltage Source  Initialize=on  Source_Type=DC  Amplitude=duty_leg_B_dc_dc_0_tx*V_dc_0_rx  Phase=0  Frequency=0  Measurements=None
  Current Measurement{,1..2,4} (4 alike) : spsCurrentMeasurementLib/Current Measurement  PhasorSimulation=off  OutputType=Complex  PSBequivalent=0
  Goto4 : Goto  Commented=on  GotoTag=v_dc_rx  TagVisibility=global
  MATLAB Function1 : MATLAB Function  TreatAsAtomicUnit=on
  MATLAB Function2 : MATLAB Function  TreatAsAtomicUnit=on
  Memory{,1..3} (4 alike) : Memory
  Product1 : Product  Inputs=3
  Product2 : Product  Inputs=3
  Series RLC Branch10 : spsSeriesRLCBranchLib/Series RLC Branch  LConnTagsString=__new0  RConnTagsString=__new0  BranchType=L  Resistance=1  Inductance=L_filtro_dc_dc  SetiL0=on  InitialCurrent=I_Lfiltro_A_0_rx  Capacitance=1e-6  Setx0=off  InitialVoltage=0  Measurements=None
  Series RLC Branch6 : spsSeriesRLCBranchLib/Series RLC Branch  LConnTagsString=__new0  RConnTagsString=__new0  BranchType=R  Resistance=Req_Lfiltro_dc_dc  Inductance=Lfiltro_dc_dc_tx  SetiL0=on  InitialCurrent=Imedia_bat_B_tx  Capacitance=1e-6  Setx0=off  InitialVoltage=0  Measurements=None
  Series RLC Branch8 : spsSeriesRLCBranchLib/Series RLC Branch  LConnTagsString=__new0  RConnTagsString=__new0  BranchType=R  Resistance=Req_Lfiltro_dc_dc  Inductance=Lfiltro_dc_dc_tx  SetiL0=on  InitialCurrent=Imedia_bat_B_tx  Capacitance=1e-6  Setx0=off  InitialVoltage=0  Measurements=None
  Series RLC Branch9 : spsSeriesRLCBranchLib/Series RLC Branch  LConnTagsString=__new0  RConnTagsString=__new0  BranchType=L  Resistance=1  Inductance=L_filtro_dc_dc  SetiL0=on  InitialCurrent=I_Lfiltro_B_0_rx  Capacitance=1e-6  Setx0=off  InitialVoltage=0  Measurements=None
  Subsystem : Subsystem  Commented=on
  Voltage Measurement : spsVoltageMeasurementLib/Voltage Measurement  Commented=on  PhasorSimulation=off  OutputType=Complex  PSBequivalent=0
  Voltage Measurement1 : spsVoltageMeasurementLib/Voltage Measurement  PhasorSimulation=off  OutputType=Complex  PSBequivalent=0
  Vdc rx : PMIOPort  Side=Left
  "Vgnd rx " : PMIOPort  Port=2  Side=Left
  Vbat + rx : PMIOPort  Port=3  Side=Right
  Vbat - rx : PMIOPort  Port=4  Side=Right
  tag scope: i_bat_rx=global, i_dc_dc_rx=global, i_leg_A_dc_dc_rx=global, i_leg_B_dc_dc_rx=global, v_bat_rx=global
  wires:
  Voltage Measurement1/1 -> [v_bat_rx]
  Voltage Measurement/1 -> Goto4/1
  Memory/1 -> Controlled Voltage Source/1
  Memory1/1 -> Controlled Voltage Source1/1
  Current Measurement4/1 -> [i_bat_rx]
  Current Measurement/1 -> [i_leg_B_dc_dc_rx]
  Memory2/1 -> Controlled Current Source2/1
  Memory3/1 -> Controlled Current Source3/1
  Current Measurement1/1 -> [i_leg_A_dc_dc_rx]
  Current Measurement2/1 -> [i_dc_dc_rx]
  [abilita_PWM_rx] -> Product1/3
  [dc_dc_leg_B_high_rx] -> Product2/1
  [dc_dc_leg_A_high_rx] -> Product1/1
  [i_leg_A_dc_dc_rx] -> Product1/2
  [abilita_PWM_rx] -> Product2/3
  [i_leg_B_dc_dc_rx] -> Product2/2
  Product2/1 -> Memory3/1
  Product1/1 -> Memory2/1
  MATLAB Function1/1(Vin) -> Memory/1
  MATLAB Function2/1(Vin) -> Memory1/1
  [v_dc_rx] -> MATLAB Function2/2(Vdc)
  [dc_dc_leg_A_high_rx] -> MATLAB Function1/5(duty)
  [dc_dc_leg_B_high_rx] -> MATLAB Function2/5(duty)
  [abilita_PWM_rx] -> MATLAB Function1/1(Abilitazione)
  [abilita_PWM_rx] -> MATLAB Function2/1(Abilitazione)
  [v_bat_rx] -> MATLAB Function1/3(Vbat)
  [v_dc_rx] -> MATLAB Function1/2(Vdc)
  [v_bat_rx] -> MATLAB Function2/3(Vbat)
  [i_leg_A_dc_dc_rx] -> MATLAB Function1/4(IL)
  [i_leg_B_dc_dc_rx] -> MATLAB Function2/4(IL)
  connections:
  Controlled Voltage Source/LConn1 -- Voltage Measurement/LConn2 -- "Vgnd rx "/RConn1 -- Controlled Current Source3/LConn1 -- Controlled Current Source2/LConn1 -- Controlled Voltage Source1/LConn1 -- Vbat - rx/RConn1 -- Voltage Measurement1/LConn2
  Voltage Measurement/LConn1 -- Current Measurement2/RConn1 -- Vdc rx/RConn1
  Current Measurement4/LConn1 -- Voltage Measurement1/LConn1 -- Vbat + rx/RConn1
  Current Measurement4/RConn1 -- Current Measurement1/LConn1 -- Current Measurement/LConn1
  Controlled Current Source3/RConn1 -- Controlled Current Source2/RConn1 -- Current Measurement2/LConn1
  Series RLC Branch6/LConn1 -- Series RLC Branch9/RConn1
  Controlled Voltage Source/RConn1 -- Series RLC Branch8/RConn1
  Current Measurement/RConn1 -- Series RLC Branch9/LConn1
  Current Measurement1/RConn1 -- Series RLC Branch10/LConn1
  Series RLC Branch10/RConn1 -- Series RLC Branch8/LConn1
  Series RLC Branch6/RConn1 -- Controlled Voltage Source1/RConn1

== system controllo_Completo_v14/Limiti Corrente Batteria rx (BMS)/Controllo carica bat tx ==
  note: Viste le convenzioni dei segni,
      | per aumentare la tensione di batteria
      |  la potenza deve essere negativa
  Vbat  rif : Inport
  Vbat : Inport  Port=2
  Ibat rif max : Inport  Port=3
  I bat rif min : Inport  Port=4
  Add : Sum  Inputs=+-
  Divide : Product  Inputs=*/
  Gain : Gain  Gain=Kp_P_tensione_batteria_rx
  Gain2 : Gain  Gain=-1
  Math Function1 : Math  Operator=square
  Math Function2 : Math  Operator=square
  "Pbat rif, Pbat max, Pbat min" : Scope  Commented=on  NumInputPorts=3
      settings: ActiveDisplayYMinimum=-6819.1166452285679  ActiveDisplayYMaximum=6819.1166452285679  DataLoggingDecimation=10  DataLoggingVariableName=ScopeData16
  Potenza Bat max : Product
  Potenza Bat min : Product
  Saturation Dynamic : simulink/Discontinuities/Saturation Dynamic  OutMin=[]  OutMax=[]  OutDataTypeStr=Inherit: Same as second input  OutDataType=fixdt(1, 16)  OutScaling=2^-10  DoSatur=off
  Ibat rif rx : Outport
  wires:
  Vbat  rif/1 -> Math Function1/1  "Vbat rif"
  Add/1 -> Gain2/1
  Gain/1 -> Saturation Dynamic/2
  Ibat rif max/1 -> Potenza Bat max/2
  Vbat/1 -> Divide/2, Potenza Bat max/1, Potenza Bat min/1, Math Function2/1  "Vbat ret"
  Potenza Bat max/1 -> "Pbat rif, Pbat max, Pbat min"/2, Saturation Dynamic/1  "Pbat max"
  I bat rif min/1 -> Potenza Bat min/2
  Potenza Bat min/1 -> "Pbat rif, Pbat max, Pbat min"/3, Saturation Dynamic/3  "Pbat min"
  Saturation Dynamic/1 -> Divide/1, "Pbat rif, Pbat max, Pbat min"/1  "Pbat rif"
  Math Function1/1 -> Add/1
  Math Function2/1 -> Add/2
  Gain2/1 -> Gain/1
  Divide/1 -> Ibat rif rx/1

== system controllo_Completo_v14/Limiti Corrente Batteria rx (BMS)/Controllo scarica bat tx ==
  note: Viste le convenzioni dei segni,
      | per aumentare la tensione di batteria
      |  la potenza deve essere negativa
  Vbat  rif : Inport
  Vbat : Inport  Port=2
  Ibat rif max : Inport  Port=3
  I bat rif min : Inport  Port=4
  Add : Sum  Inputs=+-
  Divide : Product  Inputs=*/
  Gain : Gain  Gain=Kp_P_tensione_batteria_rx
  Gain2 : Gain  Gain=-1
  Math Function1 : Math  Operator=square
  Math Function2 : Math  Operator=square
  "Pbat rif, Pbat max, Pbat min" : Scope  Commented=on  NumInputPorts=3
      settings: ActiveDisplayYMinimum=-6819.1166452285679  ActiveDisplayYMaximum=6819.1166452285679  DataLoggingDecimation=10  DataLoggingVariableName=ScopeData16
  Potenza Bat max : Product
  Potenza Bat min : Product
  Saturation Dynamic : simulink/Discontinuities/Saturation Dynamic  OutMin=[]  OutMax=[]  OutDataTypeStr=Inherit: Same as second input  OutDataType=fixdt(1, 16)  OutScaling=2^-10  DoSatur=off
  Ibat rif rx : Outport
  wires:
  Gain2/1 -> Gain/1
  Math Function2/1 -> Add/2
  Math Function1/1 -> Add/1
  Saturation Dynamic/1 -> Divide/1, "Pbat rif, Pbat max, Pbat min"/1  "Pbat rif"
  Potenza Bat min/1 -> Saturation Dynamic/3, "Pbat rif, Pbat max, Pbat min"/3  "Pbat min"
  I bat rif min/1 -> Potenza Bat min/2
  Potenza Bat max/1 -> Saturation Dynamic/1, "Pbat rif, Pbat max, Pbat min"/2  "Pbat max"
  Vbat/1 -> Divide/2, Math Function2/1, Potenza Bat min/1, Potenza Bat max/1  "Vbat ret"
  Ibat rif max/1 -> Potenza Bat max/2
  Gain/1 -> Saturation Dynamic/2
  Add/1 -> Gain2/1
  Vbat  rif/1 -> Math Function1/1  "Vbat rif"
  Divide/1 -> Ibat rif rx/1

== system controllo_Completo_v14/Limiti Corrente Batteria tx (BMS)/Controllo carica bat tx ==
  note: Viste le convenzioni dei segni,
      | per aumentare la tensione di batteria
      |  la potenza deve essere negativa
  Vbat  rif : Inport
  Vbat : Inport  Port=2
  Ibat rif max : Inport  Port=3
  I bat rif min : Inport  Port=4
  Add : Sum  Inputs=+-
  Divide : Product  Inputs=*/
  Gain : Gain  Gain=Kp_P_tensione_batteria_tx
  Gain2 : Gain  Gain=-1
  Math Function1 : Math  Operator=square
  Math Function2 : Math  Operator=square
  "Pbat rif, Pbat max, Pbat min" : Scope  Commented=on  NumInputPorts=3
      settings: ActiveDisplayYMinimum=-6819.1166452285679  ActiveDisplayYMaximum=6819.1166452285679  DataLoggingDecimation=10  DataLoggingVariableName=ScopeData16
  Potenza Bat max : Product
  Potenza Bat min : Product
  Saturation Dynamic : simulink/Discontinuities/Saturation Dynamic  OutMin=[]  OutMax=[]  OutDataTypeStr=Inherit: Same as second input  OutDataType=fixdt(1, 16)  OutScaling=2^-10  DoSatur=off
  Ibat rif tx : Outport
  wires:
  Vbat  rif/1 -> Math Function1/1  "Vbat rif"
  Add/1 -> Gain2/1
  Gain/1 -> Saturation Dynamic/2
  Ibat rif max/1 -> Potenza Bat max/2
  Vbat/1 -> Divide/2, Potenza Bat max/1, Potenza Bat min/1, Math Function2/1  "Vbat ret"
  Potenza Bat max/1 -> "Pbat rif, Pbat max, Pbat min"/2, Saturation Dynamic/1  "Pbat max"
  I bat rif min/1 -> Potenza Bat min/2
  Potenza Bat min/1 -> "Pbat rif, Pbat max, Pbat min"/3, Saturation Dynamic/3  "Pbat min"
  Saturation Dynamic/1 -> Divide/1, "Pbat rif, Pbat max, Pbat min"/1  "Pbat rif"
  Math Function1/1 -> Add/1
  Math Function2/1 -> Add/2
  Gain2/1 -> Gain/1
  Divide/1 -> Ibat rif tx/1

== system controllo_Completo_v14/Limiti Corrente Batteria tx (BMS)/Controllo scarica bat tx ==
  note: Viste le convenzioni dei segni,
      | per aumentare la tensione di batteria
      |  la potenza deve essere negativa
  Vbat  rif : Inport
  Vbat : Inport  Port=2
  Ibat rif max : Inport  Port=3
  I bat rif min : Inport  Port=4
  Add : Sum  Inputs=+-
  Divide : Product  Inputs=*/
  Gain : Gain  Gain=Kp_P_tensione_batteria_tx
  Gain2 : Gain  Gain=-1
  Math Function1 : Math  Operator=square
  Math Function2 : Math  Operator=square
  "Pbat rif, Pbat max, Pbat min" : Scope  Commented=on  NumInputPorts=3
      settings: ActiveDisplayYMinimum=-6819.1166452285679  ActiveDisplayYMaximum=6819.1166452285679  DataLoggingDecimation=10  DataLoggingVariableName=ScopeData16
  Potenza Bat max : Product
  Potenza Bat min : Product
  Saturation Dynamic : simulink/Discontinuities/Saturation Dynamic  OutMin=[]  OutMax=[]  OutDataTypeStr=Inherit: Same as second input  OutDataType=fixdt(1, 16)  OutScaling=2^-10  DoSatur=off
  Ibat rif tx : Outport
  wires:
  Gain2/1 -> Gain/1
  Math Function2/1 -> Add/2
  Math Function1/1 -> Add/1
  Saturation Dynamic/1 -> Divide/1, "Pbat rif, Pbat max, Pbat min"/1  "Pbat rif"
  Potenza Bat min/1 -> Saturation Dynamic/3, "Pbat rif, Pbat max, Pbat min"/3  "Pbat min"
  I bat rif min/1 -> Potenza Bat min/2
  Potenza Bat max/1 -> Saturation Dynamic/1, "Pbat rif, Pbat max, Pbat min"/2  "Pbat max"
  Vbat/1 -> Divide/2, Math Function2/1, Potenza Bat min/1, Potenza Bat max/1  "Vbat ret"
  Ibat rif max/1 -> Potenza Bat max/2
  Gain/1 -> Saturation Dynamic/2
  Add/1 -> Gain2/1
  Vbat  rif/1 -> Math Function1/1  "Vbat rif"
  Divide/1 -> Ibat rif tx/1

== system controllo_Completo_v14/Visualizzazione/Subsystem ==
  i bat tx : Inport
  v bat tx : Inport  Port=2
  i bat rx : Inport  Port=3
  v bat rx : Inport  Port=4
  Abs : Abs  SaturateOnIntegerOverflow=off
  Abs1 : Abs  SaturateOnIntegerOverflow=off
  Divide : Product  Inputs=*/
  Divide1 : Product  Inputs=*/
  MinMax : MinMax  Inputs=2
  Mux10 : Mux  Inputs=2
  Product : Product
  Product1 : Product
  Saturation1 : Saturate  UpperLimit=inf  LowerLimit=1
  Saturation2 : Saturate  UpperLimit=1  LowerLimit=0
  Saturation3 : Saturate  UpperLimit=1  LowerLimit=0
  Saturation4 : Saturate  UpperLimit=inf  LowerLimit=1
  "P tx, Prx" : Outport
  eta : Outport  Port=2
  wires:
  Saturation1/1 -> Divide1/2
  Saturation4/1 -> Divide/2
  MinMax/1 -> eta/1
  v bat tx/1 -> Product/2
  Mux10/1 -> "P tx, Prx"/1
  i bat tx/1 -> Product/1
  Saturation3/1 -> MinMax/2
  Abs/1 -> Mux10/1, Divide/1, Saturation1/1
  Saturation2/1 -> MinMax/1
  Divide/1 -> Saturation2/1
  v bat rx/1 -> Product1/2
  Product1/1 -> Abs1/1
  Product/1 -> Abs/1
  Abs1/1 -> Mux10/2, Divide1/1, Saturation4/1
  i bat rx/1 -> Product1/1
  Divide1/1 -> Saturation3/1

== system controllo_Completo_v14/Controllo  rx/Modulazione PS/Dead time ==
  high A : Inport
  low A : Inport  Port=2
  high B : Inport  Port=3
  low B : Inport  Port=4
  dead time : Subsystem  VariantControl=Selettore_No_Dead_Time_0_Dead_Time_1_rx==1
  no dead time : Subsystem  VariantControl=Selettore_No_Dead_Time_0_Dead_Time_1_rx==0
  high A DT : Outport
  low A DT : Outport  Port=2
  high B DT : Outport  Port=3
  low B DT : Outport  Port=4

== system controllo_Completo_v14/Controllo  rx/Modulazione PS/Phase shift ==
  duty A : Inport
  duty B : Inport  Port=2
  abilita PWM : Inport  Port=3
  Fronte Discesa : Subsystem
  "Fronte Discesa " : Subsystem
  Fronte Salita : Subsystem
  "Fronte Salita " : Subsystem
  Logical Operator{,1..3} (4 alike) : Logic  AllPortsSameDT=off  OutDataTypeStr=boolean
  Relational Operator : RelationalOperator  OutDataTypeStr=boolean  RndMeth=Simplest  InputSameDT=off
  Relational Operator1 : RelationalOperator  OutDataTypeStr=boolean  RndMeth=Simplest  InputSameDT=off
  Repeating Sequence : simulink/Sources/Repeating Sequence  rep_seq_t=[0 1/2 1]*T_dc_ac  rep_seq_y=[1 0 1]
  Repeating Sequence1 : simulink/Sources/Repeating Sequence  rep_seq_t=[0 1/2 1]*T_dc_ac  rep_seq_y=[1 0 1]
  S-R Flip-Flop2 : simulink_extras/Flip Flops/S-R Flip-Flop  initial_condition=0
  S-R Flip-Flop3 : simulink_extras/Flip Flops/S-R Flip-Flop  initial_condition=0
  high A : Outport
  low A : Outport  Port=2
  high B : Outport  Port=3
  low B : Outport  Port=4
  wires:
  Repeating Sequence/1 -> Relational Operator/2
  duty B/1 -> Relational Operator1/1
  Relational Operator/1 -> "Fronte Discesa "/1(In1), Fronte Salita/1(In1)
  Relational Operator1/1 -> "Fronte Salita "/1(In1), Fronte Discesa/1(In1)
  Repeating Sequence1/1 -> Relational Operator1/2
  duty A/1 -> Relational Operator/1
  Fronte Salita/1(Out1) -> S-R Flip-Flop2/1
  Fronte Discesa/1(Out1) -> S-R Flip-Flop2/2
  S-R Flip-Flop2/1 -> Logical Operator/1
  S-R Flip-Flop2/2 -> Logical Operator1/1
  "Fronte Salita "/1(Out1) -> S-R Flip-Flop3/1
  "Fronte Discesa "/1(Out1) -> S-R Flip-Flop3/2
  S-R Flip-Flop3/1 -> Logical Operator2/1
  S-R Flip-Flop3/2 -> Logical Operator3/1
  Logical Operator/1 -> high A/1
  Logical Operator1/1 -> low A/1
  Logical Operator2/1 -> high B/1
  Logical Operator3/1 -> low B/1
  abilita PWM/1 -> Logical Operator3/2, Logical Operator2/2, Logical Operator1/2, Logical Operator/2

== system controllo_Completo_v14/Controllo  rx/Modulazione PWM/Variant Subsystem ==
  high A : Inport
  low A : Inport  Port=2
  high B : Inport  Port=3
  low B : Inport  Port=4
  dead time : Subsystem  VariantControl=(Selettore_No_Dead_Time_0_Dead_Time_1_rx==1)&(Selettore_Switching_0_Valori_Medi_1_dc_dc_rx==0)
  no dead time : Subsystem  VariantControl=(Selettore_No_Dead_Time_0_Dead_Time_1_rx==0)|(Selettore_Switching_0_Valori_Medi_1_dc_dc_rx==1)
  high A DT : Outport
  low A DT : Outport  Port=2
  high B DT : Outport  Port=3
  low B DT : Outport  Port=4

== system controllo_Completo_v14/Controllo  rx/Modulazione PWM/Variant Subsystem1 ==
  duty A : Inport
  duty B : Inport  Port=2
  abilita PWM : Inport  Port=3
  Modulazione Lineare : Subsystem  VariantControl=Selettore_Switching_0_Valori_Medi_1_dc_dc_rx==1
  PWM Seno-Triangolo : Subsystem  VariantControl=Selettore_Switching_0_Valori_Medi_1_dc_dc_rx==0
  high A : Outport
  low A : Outport  Port=2
  high B : Outport  Port=3
  low B : Outport  Port=4

== system controllo_Completo_v14/Controllo tx/Modulazione PS/Dead time ==
  high A : Inport
  low A : Inport  Port=2
  high B : Inport  Port=3
  low B : Inport  Port=4
  dead time : Subsystem  VariantControl=Selettore_No_Dead_Time_0_Dead_Time_1_tx==1
  no dead time : Subsystem  VariantControl=Selettore_No_Dead_Time_0_Dead_Time_1_tx==0
  high A DT : Outport
  low A DT : Outport  Port=2
  high B DT : Outport  Port=3
  low B DT : Outport  Port=4
